simulink model "Load_torque_estimator"  (R2021a)
settings: Solver=VariableStepAuto  StartTime=0.0  StopTime=10.0  RelTol=1e-3
settings Model: Creator=Mehra  LastModifiedBy=Mehra

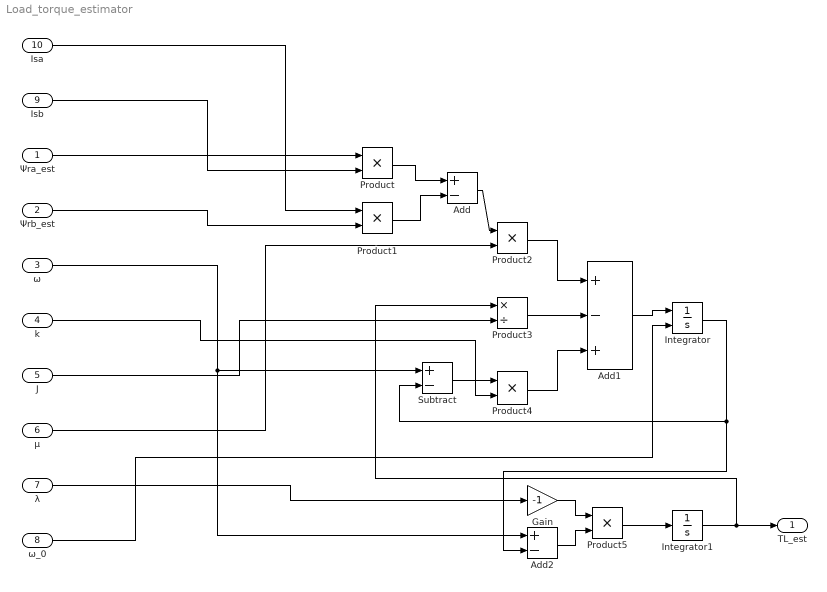
== system Load_torque_estimator ==
  Ψra_est : Inport
  Ψrb_est : Inport  Port=2
  ω : Inport  Port=3
  k : Inport  Port=4
  J : Inport  Port=5
  µ : Inport  Port=6
  λ : Inport  Port=7
  ω_0 : Inport  Port=8
  Isb : Inport  Port=9
  Isa : Inport  Port=10
  Add : Sum  Inputs=+-
  Add1 : Sum  Inputs=+-+
  Add2 : Sum  Inputs=+-
  Gain : Gain  Gain=-1
  Integrator : Integrator  InitialConditionSource=external
  Integrator1 : Integrator
  Product{,1..2,4..5} (5 alike) : Product
  Product3 : Product  Inputs=*/
  Subtract : Sum  Inputs=+-
  TL_est : Outport
  wires:
  Product/1 -> Add/1
  Product1/1 -> Add/2
  Add/1 -> Product2/1
  µ/1 -> Product2/2
  J/1 -> Product3/2
  Subtract/1 -> Product4/1
  ω/1 -> Add2/1, Subtract/1
  k/1 -> Product4/2
  Product2/1 -> Add1/1
  Product3/1 -> Add1/2
  Product4/1 -> Add1/3
  Add2/1 -> Product5/2
  Gain/1 -> Product5/1
  λ/1 -> Gain/1
  Add1/1 -> Integrator/1
  ω_0/1 -> Integrator/2
  Integrator/1 -> Subtract/2, Add2/2
  Product5/1 -> Integrator1/1
  Integrator1/1 -> Product3/1, TL_est/1
  Ψra_est/1 -> Product/1
  Isb/1 -> Product/2
  Ψrb_est/1 -> Product1/2
  Isa/1 -> Product1/1
